simulink library "IIT_Genoa_Intan_HDL_blocks"  (R2020a)
settings: Solver=VariableStepAuto  StartTime=0.0  StopTime=10.0  RelTol=1e-3
libraries: simulink x93, hdlsllib x68
(part 1 of 3)
settings Model: Creator=diflo  LastModifiedBy=diflo

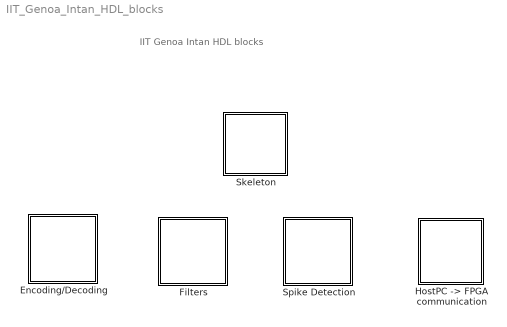
== system IIT_Genoa_Intan_HDL_blocks ==
  note: IIT Genoa Intan HDL blocks
  Encoding/Decoding : Subsystem
  Filters : Subsystem
  "HostPC -> FPGA communication" : Subsystem
  Skeleton : Subsystem
  Spike Detection : Subsystem

== system IIT_Genoa_Intan_HDL_blocks/Encoding//Decoding ==
  input_interpret_store_retrieve : Subsystem
      mask DialogControl DescGroupVar Prompt: Decoding subsystem
      mask DialogControl DescTextVar Prompt: This subsystem interprets the retrieved data from the Finite State Machine of the Intan RHS by assigning a specific value according to the data type.
      mask Display:
      | color('white'); port_label('input',1,'FIFO_data_in')
      | color('white'); port_label('input',2,'FIFO_write_to')
      | color('white'); port_label('input',3,'read_output_data_input_interpret_store_retrieve')
      | color('white'); port_label('input',4,'data_stream_enable')
      | color('white'); port_label('output',1,'InputState')
      | color('white'); port_label('output',2,'output_data_input_interpret_store_retrieve')
      | color('white'); port_label('output',3,'output_data_to_process')
      | color('white'); port_label('output',4,'address_output_data_to_process')
  output_interpret_collect_output : Subsystem
      mask DialogControl DescGroupVar Prompt: Encoding subsystem
      mask DialogControl DescTextVar Prompt: This subsystem reconstructs the logic of the dataflow in order to send the data to the Host PC.
      mask Display:
      | color('white'); port_label('input',1,'FIFO_data_in')
      | color('white'); port_label('input',2,'FIFO_write_to')
      | color('white'); port_label('input',3,'InputState')
      | color('white'); port_label('input',4,'data_stream_enable')
      | color('white'); port_label('input',5,'output_data_input_interpret_store_retrieve')
      | color('white'); port_label('input',6,'filter_output_or_spike')
      | color('white'); port_label('output',1,'comp_data_out_valid')
      | color('white'); port_label('output',2,'comp_data_out')
      | color('white'); port_label('output',3,'read_filter_output_or_spike')
      | color('white'); port_label('output',4,'OutputState')
      | color('white'); port_label('output',5,'read_output_data_input_interpret_store_retrieve')

== system IIT_Genoa_Intan_HDL_blocks/Filters ==
  Butter_1st_HP : Subsystem  mask{s1=0.969531252908746199, a21=-0.939062505817492399}
      mask DialogControl DescGroupVar Prompt: Direct Form II - Butterworth 1st Order HP filter
      mask DialogControl DescTextVar Prompt: Butterworth 1st order highpass filtering logic. The filter is fully serial implemented with a custom architecture according to the logic of the input dataflow from the Finite State Machine of the Intan RHS.
      mask DialogControl Container3 Prompt: Filter coefficients
      mask Display:
      | color('white'); port_label('input',1,'output_data_to_process')
      | color('white'); port_label('input',2,'InputState')
      | color('white'); port_label('input',3,'address_output_data_to_process')
      | color('white'); port_label('input',4,'read_filter_output_or_spike')
      | color('white'); port_label('output',1,'filter_output')
      | color('white'); port_label('output',2,'filter_writing_address')
      | color('white'); port_label('output',3,'filter_writing_enable')
      | color('white'); port_label('output',4,'filter_output_or_spike')
  Butter_2nd_HP : Subsystem  mask{s1=0.956543225556876764, a21=-1.9111970674260732, a31=0.914975834801433852, b21=-2}
      mask DialogControl DescGroupVar Prompt: Direct Form II - Butterworth 2nd Order HP filter
      mask DialogControl DescTextVar Prompt: Butterworth 2nd order highpass filtering logic. The filter is fully serial implemented with a custom architecture according to the logic of the input dataflow from the Finite State Machine of the Intan RHS.
      mask DialogControl ParameterGroupVar Prompt: Filter coefficients
      mask Display:
      | color('white'); port_label('input',1,'output_data_to_process')
      | color('white'); port_label('input',2,'InputState')
      | color('white'); port_label('input',3,'address_output_data_to_process')
      | color('white'); port_label('input',4,'read_filter_output_or_spike')
      | color('white'); port_label('output',1,'filter_output')
      | color('white'); port_label('output',2,'filter_writing_address')
      | color('white'); port_label('output',3,'filter_writing_enable')
      | color('white'); port_label('output',4,'filter_output_or_spike')

== system IIT_Genoa_Intan_HDL_blocks/HostPC -> FPGA communication ==
  interpret_pipe_in : Subsystem  TreatAsAtomicUnit=on
      mask DialogControl DescGroupVar Prompt: Pipe in interpret
      mask DialogControl DescTextVar Prompt: This subsystem interprets the configuration file loaded by the GUI running in the Host PC. It is possible to communicate a single value of threshold and refractory period for all the channels.
      mask Display:
      | color('white'); port_label('input',1,'pipe_in_data')
      | color('white'); port_label('output',1,'pipe_in_threshold')
      | color('white'); port_label('output',2,'pipe_in_refractory')

== system IIT_Genoa_Intan_HDL_blocks/Skeleton ==
  cust_architecture : Subsystem
      mask DialogControl DescGroupVar Prompt: Custom Architecture Skeleton
      mask DialogControl DescTextVar Prompt: High level skeleton of the custom architecture. The entire algorithm must be developed inside this subsystem.
      mask Display:
      | color('white'); port_label('input',1,'FIFO_data_in')
      | color('white'); port_label('input',2,'FIFO_write_to')
      | color('white'); port_label('input',3,'data_stream_enable')
      | color('white'); port_label('input',4,'pipe_in_data')
      | color('white'); port_label('input',5,'pipe_in_en')
      | color('white'); port_label('input',6,'pipe_out_read')
      | color('white'); port_label('input',7,'cfg')
      | color('white'); port_label('output',1,'comp_data_out')
      | color('white'); port_label('output',2,'comp_data_out_valid')
      | color('white'); port_label('output',3,'trig_stim')
      | color('white'); port_label('output',4,'computing')
      | color('white'); port_label('output',5,'pipe_out_data')
      | color('white'); port_label('output',6,'status')

== system IIT_Genoa_Intan_HDL_blocks/Spike Detection ==
  General : Subsystem
  Sample Thresholding : Subsystem
  Sample Trhesholding pipe in : Subsystem

== system IIT_Genoa_Intan_HDL_blocks/Encoding//Decoding/input_interpret_store_retrieve ==
  note: data sent to Output
  note: data sent for processing
  note: address sent for processing
  note: reading address
      | from output
  FIFO_data_in : Inport
  FIFO_write_to : Inport  Port=2
  read_output_data_input_interpret_store_retrieve : Inport  Port=3
  data_stream_enable : Inport  Port=4
  InputStateMachine : Stateflow chart  TreatAsAtomicUnit=on
  Interpret_to_RAM_input : Subsystem
  store_and_retrieve_input : Subsystem
  InputState : Outport
  output_data_input_interpret_store_retrieve : Outport  Port=2
  output_data_to_process : Outport  Port=3
  address_output_data_to_process : Outport  Port=4
  wires:
  Interpret_to_RAM_input/4(write address) -> store_and_retrieve_input/3(wr_address)
  Interpret_to_RAM_input/5(wr_en) -> store_and_retrieve_input/4(wr_en)
  InputStateMachine/1(InputState) -> store_and_retrieve_input/5(InputState), InputState/1, Interpret_to_RAM_input/3(InputState)  "InputState"
  store_and_retrieve_input/1(read_from_storage_value) -> output_data_input_interpret_store_retrieve/1
  Interpret_to_RAM_input/2(inc_source_device) -> InputStateMachine/4(inc_source_device_MSB)
  Interpret_to_RAM_input/1(device_output) -> InputStateMachine/3(channel_0_19)
  Interpret_to_RAM_input/3(wr_din) -> store_and_retrieve_input/2(wr_din)
  FIFO_data_in/1 -> InputStateMachine/1(FIFO_data_in), Interpret_to_RAM_input/1(FIFO_data_in)
  FIFO_write_to/1 -> Interpret_to_RAM_input/2(FIFO_write_to), InputStateMachine/2(FIFO_write_to)
  read_output_data_input_interpret_store_retrieve/1 -> store_and_retrieve_input/1(read address)
  data_stream_enable/1 -> Interpret_to_RAM_input/4(data_stream_enable)
  store_and_retrieve_input/3(read_from_porcessing_addr) -> address_output_data_to_process/1
  store_and_retrieve_input/2(current_value) -> output_data_to_process/1

== system IIT_Genoa_Intan_HDL_blocks/Encoding//Decoding/output_interpret_collect_output ==
  FIFO_data_in : Inport
  FIFO_write_to : Inport  Port=2
  InputState : Inport  Port=3
  data_stream_enable : Inport  Port=4
  output_data_input_interpret_store_retrieve : Inport  Port=5
  filter_output_or_spike : Inport  Port=6
  collect_output : Subsystem
  output_interpret : Subsystem
  comp_data_out_valid : Outport
  comp_data_out : Outport  Port=2
  read_filter_output_or_spike : Outport  Port=3
  OutputState : Outport  Port=4
  read_output_data_input_interpret_store_retrieve : Outport  Port=5
  wires:
  FIFO_data_in/1 -> collect_output/1(FIFO_data_in)
  output_interpret/1(OutputState) -> OutputState/1, collect_output/4(OutputState)
  FIFO_write_to/1 -> collect_output/2(FIFO_write_to)
  collect_output/2(comp_data_out) -> comp_data_out/1
  output_interpret/2(rd_enable) -> collect_output/5(rd_enable)
  output_interpret/3(read_output_data_input_interpret_store_retrieve) -> read_output_data_input_interpret_store_retrieve/1, collect_output/6(rd_address)
  collect_output/1(comp_data_out_valid) -> comp_data_out_valid/1
  output_data_input_interpret_store_retrieve/1 -> collect_output/7(read_from_storage_value)
  collect_output/3(rd_address_bit_set_AC_during_DC) -> read_filter_output_or_spike/1
  filter_output_or_spike/1 -> collect_output/8(rd_dout)
  data_stream_enable/1 -> output_interpret/1(data_stream_enable)
  InputState/1 -> output_interpret/2(InputState), collect_output/3(InputState)

== system IIT_Genoa_Intan_HDL_blocks/Filters/Butter_1st_HP ==
  output_data_to_process : Inport
  InputState : Inport  Port=2
  address_output_data_to_process : Inport  Port=3
  read_filter_output_or_spike : Inport  Port=4
  ProcessedData_storage : hdlsllib/HDL RAMs/Dual Port RAM  ram_size=9
      settings: SourceProductBaseCode=SL
  Subsystem : Subsystem
  Terminator1 : Terminator
  filter_output : Outport
  filter_writing_address : Outport  Port=2
  filter_writing_enable : Outport  Port=3
  filter_output_or_spike : Outport  Port=4
  wires:
  ProcessedData_storage/1 -> Terminator1/1
  ProcessedData_storage/2 -> filter_output_or_spike/1  "filtered_sample"
  read_filter_output_or_spike/1 -> ProcessedData_storage/4
  Subsystem/1(filter_output) -> filter_output/1, ProcessedData_storage/1
  Subsystem/2(filter_writing_address) -> filter_writing_address/1, ProcessedData_storage/2
  output_data_to_process/1 -> Subsystem/1(output_data_to_process)
  InputState/1 -> Subsystem/2(InputState)
  address_output_data_to_process/1 -> Subsystem/3(address_output_data_to_process)
  Subsystem/3(filter_writing_enable) -> filter_writing_enable/1, ProcessedData_storage/3

== system IIT_Genoa_Intan_HDL_blocks/Filters/Butter_2nd_HP ==
  output_data_to_process : Inport
  InputState : Inport  Port=2
  address_output_data_to_process : Inport  Port=3
  read_filter_output_or_spike : Inport  Port=4
  ProcessedData_storage : hdlsllib/HDL RAMs/Dual Port RAM  ram_size=9
      settings: SourceProductBaseCode=SL
  Terminator7 : Terminator
  filtering : Subsystem
  filter_output : Outport
  filter_writing_address : Outport  Port=2
  filter_writing_enable : Outport  Port=3
  filter_output_or_spike : Outport  Port=4
  wires:
  filtering/2(filter_writing_address) -> filter_writing_address/1, ProcessedData_storage/2
  filtering/3(filter_writing_enable) -> filter_writing_enable/1, ProcessedData_storage/3
  InputState/1 -> filtering/2(InputState)
  ProcessedData_storage/1 -> Terminator7/1
  read_filter_output_or_spike/1 -> ProcessedData_storage/4
  filtering/1(filter_output) -> filter_output/1, ProcessedData_storage/1
  output_data_to_process/1 -> filtering/1(output_data_to_process)
  ProcessedData_storage/2 -> filter_output_or_spike/1
  address_output_data_to_process/1 -> filtering/3(address_output_data_to_process)

== system IIT_Genoa_Intan_HDL_blocks/HostPC -> FPGA communication/interpret_pipe_in ==
  pipe_in_data : Inport
  pipe_in_refractory : Subsystem
  pipe_in_th : Subsystem
  threshold : Outport
  refractory : Outport  Port=2
  wires:
  pipe_in_data/1 -> pipe_in_th/1(value_from_pipe_in), pipe_in_refractory/1(value_from_pipe_in)
  pipe_in_refractory/1(refractory) -> refractory/1
  pipe_in_th/1(th) -> threshold/1

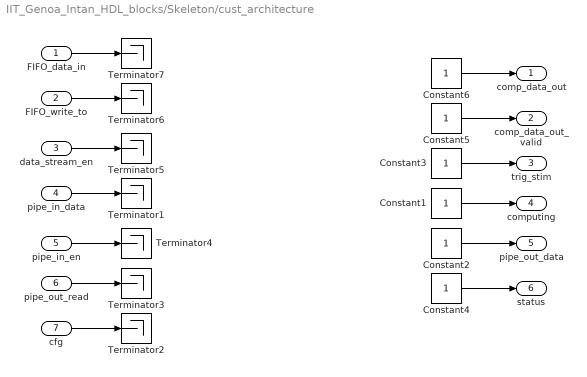
== system IIT_Genoa_Intan_HDL_blocks/Skeleton/cust_architecture ==
  FIFO_data_in : Inport
  FIFO_write_to : Inport  Port=2
  data_stream_en : Inport  Port=3
  pipe_in_data : Inport  Port=4
  pipe_in_en : Inport  Port=5
  pipe_out_read : Inport  Port=6
  cfg : Inport  Port=7
  Constant{1..6} (6 alike) : Constant  OutDataTypeStr=uint16  SampleTime=-1
  Terminator{1..7} (7 alike) : Terminator
  comp_data_out : Outport  VectorParamsAs1DForOutWhenUnconnected=off
  comp_data_out_valid : Outport  Port=2  OutDataTypeStr=boolean  VectorParamsAs1DForOutWhenUnconnected=off
  trig_stim : Outport  Port=3  VectorParamsAs1DForOutWhenUnconnected=off
  computing : Outport  Port=4  VectorParamsAs1DForOutWhenUnconnected=off
  pipe_out_data : Outport  Port=5  VectorParamsAs1DForOutWhenUnconnected=off
  status : Outport  Port=6  VectorParamsAs1DForOutWhenUnconnected=off
  wires:
  Constant3/1 -> trig_stim/1
  Constant1/1 -> computing/1
  Constant2/1 -> pipe_out_data/1
  Constant4/1 -> status/1
  cfg/1 -> Terminator2/1
  pipe_out_read/1 -> Terminator3/1
  pipe_in_en/1 -> Terminator4/1
  data_stream_en/1 -> Terminator5/1
  FIFO_write_to/1 -> Terminator6/1
  pipe_in_data/1 -> Terminator1/1
  FIFO_data_in/1 -> Terminator7/1
  Constant5/1 -> comp_data_out_valid/1
  Constant6/1 -> comp_data_out/1

== system IIT_Genoa_Intan_HDL_blocks/Spike Detection/General ==
  processing_output_logic : Subsystem
      mask DialogControl DescGroupVar Prompt: Output logic Filter/Spike Detection
      mask DialogControl DescTextVar Prompt: This subsystem is needed in order to send to the Host PC at the right time the filter outputs and the detected spikes
      mask Display:
      | color('white'); port_label('input',1,'OutputState')
      | color('white'); port_label('input',2,'filter_output')
      | color('white'); port_label('input',3,'spike')
      | color('white'); port_label('output',1,'to_output_interpret_collect_output')
  refractory_period : Subsystem  mask{refractory=0}
      mask prompts: refractory "Refractory period (samples)"
      mask DialogControl DescGroupVar Prompt: Refractory period
      mask DialogControl DescTextVar Prompt: Subsystem to compute the refractory period.
      mask Display:
      | color('white'); port_label('input',1,'filter_writing_enable')
      | color('white'); port_label('input',2,'spike_check')
      | color('white'); port_label('input',3,'filter_writing_address')
      | color('white'); port_label('input',4,'read_filter_output_or_spike')
      | color('white'); port_label('output',1,'refractory_check')
      | color('white'); port_label('output',2,'spike')
  refractory_period_pipe_in : Subsystem  AncestorBlock=IIT_Genoa_Intan_HDL_blocks/refractory_period
      mask DialogControl DescGroupVar Prompt: Refractory period (pipe in)
      mask DialogControl DescTextVar Prompt: Subsystem to compute the refractory period. The refractory period can be selected loading a configuration file from the GUI running in the Host PC in order to change in real time the value. This subsystem allows to set a single refractory period for all the channels.
      mask Display:
      | color('white'); port_label('input',1,'filter_writing_enable')
      | color('white'); port_label('input',2,'spike_check')
      | color('white'); port_label('input',3,'filter_writing_address')
      | color('white'); port_label('input',4,'read_filter_output_or_spike')
      | color('white'); port_label('input',5,'pipe_in_refractory')
      | color('white'); port_label('output',1,'refractory_check')
      | color('white'); port_label('output',2,'spike')
  spike_check : Subsystem
      mask DialogControl DescGroupVar Prompt: Spike check
      mask DialogControl DescTextVar Prompt: The ouput of this subsystem is 1 if both the refractory period condition and the amplitude check are TRUE, thus, a spike is detected and its timestamp stored.
      mask Display:
      | color('white'); port_label('input',1,'detection_check')
      | color('white'); port_label('input',2,'refractory_check')
      | color('white'); port_label('output',1,'spike_check')

== system IIT_Genoa_Intan_HDL_blocks/Spike Detection/Sample Thresholding ==
  HardThreshold : Subsystem  mask{th=0}
      mask prompts: th "Threshold (µV)"
      mask DialogControl DescGroupVar Prompt: Hard Threshold
      mask DialogControl DescTextVar Prompt: This subsystem computes a spike detection based on the identification of a sample in the signal below a set threshold. It detects as a potential each sample below threshold
      mask DialogControl ParameterGroupVar Prompt: Spike Detection Parametes
      mask Display:
      | color('white'); port_label('input',1,'filter_output')
      | color('white'); port_label('output',1,'detection_check')
  LocalMaxima : Subsystem  mask{th=0}
      mask prompts: th "Threshold (µV)"
      mask DialogControl DescGroupVar Prompt: Hard Threshold Local Maxima
      mask DialogControl DescTextVar Prompt: This subsystem computes a spike detection based on the identification of a peak in the signal below a set threshold. It takes into account the samples at time t, t-1 and t-2 to detect a potential negative peak below threshold.
      mask DialogControl Container Prompt: Spike detection parameters
      mask Display:
      | color('white'); port_label('input',1,'filter_output')
      | color('white'); port_label('input',2,'filter_writing_enable')
      | color('white'); port_label('input',3,'filter_writing_address')
      | color('white'); port_label('output',1,'detection_check')

== system IIT_Genoa_Intan_HDL_blocks/Spike Detection/Sample Trhesholding pipe in ==
  HardThreshold_pipein : Subsystem  AncestorBlock=IIT_Genoa_Intan_HDL_blocks/HardThreshold
      mask DialogControl DescGroupVar Prompt: Hard Threshold
      mask DialogControl DescTextVar Prompt: This subsystem computes a spike detection based on the identification of a sample in the signal below a set threshold. It detects as a potential each sample below threshold. The threshold can be selected loading a configuration file from the GUI running in the Host PC in order to change in real time the value. This subsystem allows to set a single threshold for all the channels.
      mask Display:
      | color('white'); port_label('input',1,'filter_output')
      | color('white'); port_label('input',2,'pipe_in_threshold')
      | color('white'); port_label('output',1,'detection_check')
  LocalMaxima_pipein : Subsystem  AncestorBlock=IIT_Genoa_Intan_HDL_blocks/LocalMaxima
      mask DialogControl DescGroupVar Prompt: Hard Threshold Local Maxima (pipe in)
      mask DialogControl DescTextVar Prompt: This subsystem computes a spike detection based on the identification of a peak in the signal below a set threshold. It takes into account the samples at time t, t-1 and t-2 to detect a potential negative peak below threshold. The threshold can be selected loading a configuration file from the GUI running in the Host PC in order to change in real time the value. This subsystem allows to set a single threshold for all the channels.
      mask Display:
      | color('white'); port_label('input',1,'filter_output')
      | color('white'); port_label('input',2,'filter_writing_enable')
      | color('white'); port_label('input',3,'filter_writing_address')
      | color('white'); port_label('input',4,'pipe_in_threshold')
      | color('white'); port_label('output',1,'detection_check')

== system IIT_Genoa_Intan_HDL_blocks/Encoding//Decoding/input_interpret_store_retrieve/Interpret_to_RAM_input ==
  note: These subsystems identify the sources of the incoming data (amplifier --> source_device and channel number) and
      | determine the address to be associated to the current data for the RAM storage. This statement is valid for all the kind of
      | data except for the magic number and the timestamp that are directly sent to a different RAM in the Output section
  FIFO_data_in : Inport
  FIFO_write_to : Inport  Port=2
  InputState : Inport  Port=3
  data_stream_enable : Inport  Port=4
  RAM address definition : Subsystem
  interpret incoming data : Subsystem
  device_output : Outport
  inc_source_device : Outport  Port=2
  wr_din : Outport  Port=3
  write address : Outport  Port=4
  wr_en : Outport  Port=5
  wires:
  interpret incoming data/4(source_channel_0_159) -> RAM address definition/3(source_channel_0_159)
  interpret incoming data/2(inc_source_device) -> inc_source_device/1
  interpret incoming data/1(source_device) -> RAM address definition/4(source_device)
  data_stream_enable/1 -> interpret incoming data/3(data_stream_enable)
  RAM address definition/3(write_enable_6to15) -> wr_en/1  "wr_en"
  interpret incoming data/3(device_output) -> device_output/1
  InputState/1 -> RAM address definition/2(InputState), interpret incoming data/2(InputState)
  interpret incoming data/5(converter_cnt) -> RAM address definition/5(converter_cnt)
  FIFO_write_to/1 -> RAM address definition/6(write_to), interpret incoming data/1(FIFO_write_to)
  FIFO_data_in/1 -> RAM address definition/1(DataIn)
  RAM address definition/2(wr_addr) -> write address/1  "write address"
  RAM address definition/1(wr_din) -> wr_din/1  "wr_din"

== system IIT_Genoa_Intan_HDL_blocks/Encoding//Decoding/input_interpret_store_retrieve/store_and_retrieve_input ==
  note: Two dual-port RAM for storage and processing
  note: current data
  note: data sent to Output
  note: data sent for processing
  note: this memory is for synchronizing the current value and
      | the read_from_porcessing_addr since to ouput a value
      | the dual port RAM needs a single clock
  note: current data
  note: reading address
      | from output
  note: address sent for processing
  note: writing address
  read address : Inport
  wr_din : Inport  Port=2
  wr_address : Inport  Port=3
  wr_en : Inport  Port=4
  InputState : Inport  Port=5
  Compare To Constant : simulink/Logic and Bit Operations/Compare To Constant  relop===  const=7  OutDataTypeStr=boolean
  Delay1 : Delay  DelayLength=1  InitialCondition=0
  Terminator : Terminator
  Terminator6 : Terminator
  input_storage : hdlsllib/HDL RAMs/Dual Port RAM  ram_size=9
      settings: SourceProductBaseCode=SL
  input_storage_for_processing : hdlsllib/HDL RAMs/Dual Port RAM  ram_size=9
      settings: SourceProductBaseCode=SL
  read_from_storage_value : Outport
  current_value : Outport  Port=2
  read_from_porcessing_addr : Outport  Port=3
  wires:
  wr_en/1 -> input_storage/3
  InputState/1 -> Compare To Constant/1
  Compare To Constant/1 -> input_storage_for_processing/3
  input_storage_for_processing/2 -> current_value/1  "current value"
  Delay1/1 -> read_from_porcessing_addr/1, input_storage_for_processing/4  "read from porcessing addr"
  input_storage/1 -> Terminator/1
  wr_address/1 -> Delay1/1, input_storage_for_processing/2, input_storage/2
  wr_din/1 -> input_storage_for_processing/1, input_storage/1
  input_storage/2 -> read_from_storage_value/1  "read_from_storage"
  input_storage_for_processing/1 -> Terminator6/1
  read address/1 -> input_storage/4

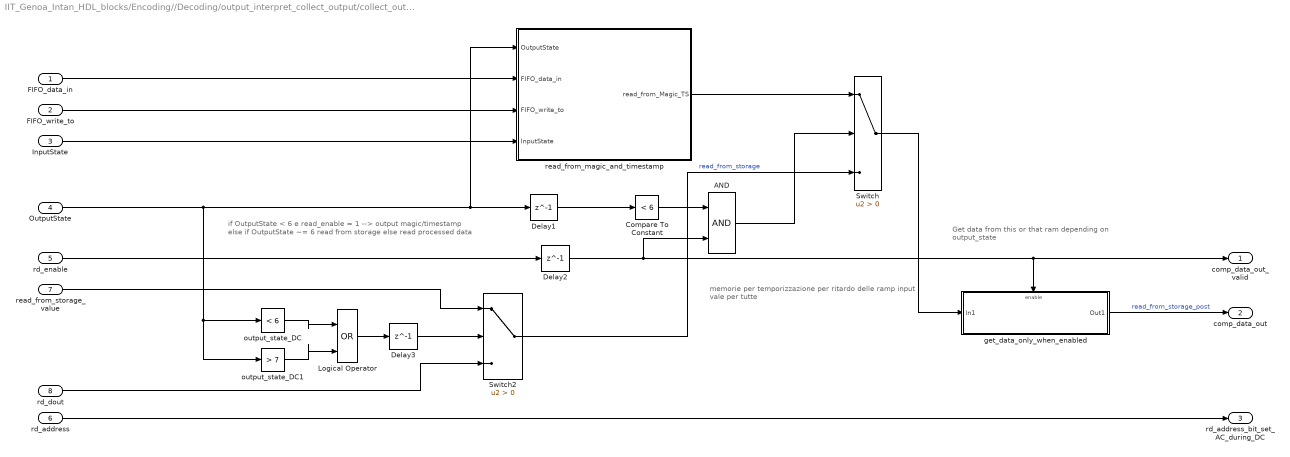
== system IIT_Genoa_Intan_HDL_blocks/Encoding//Decoding/output_interpret_collect_output/collect_output ==
  note: if OutputState < 6 e read_enable = 1 --> output magic/timestamp
      | else if OutputState ~= 6 read from storage
      | else read processed data
  note: memorie per temporizzazione per ritardo delle ramp input
      | vale per tutte
  note: Get data from this or that ram depending on output_state
  FIFO_data_in : Inport
  FIFO_write_to : Inport  Port=2
  InputState : Inport  Port=3
  OutputState : Inport  Port=4
  rd_enable : Inport  Port=5
  rd_address : Inport  Port=6
  read_from_storage_value : Inport  Port=7
  rd_dout : Inport  Port=8
  AND : Logic  IconShape=distinctive  AllPortsSameDT=off  OutDataTypeStr=boolean
  Compare To Constant : simulink/Logic and Bit Operations/Compare To Constant  relop=<  const=6  OutDataTypeStr=boolean
  Delay1 : Delay  DelayLength=1  InitialCondition=0
  Delay2 : Delay  DelayLength=1  InitialCondition=0
  Delay3 : Delay  DelayLength=1  InitialCondition=0
  Logical Operator : Logic  Operator=OR  IconShape=distinctive  AllPortsSameDT=off  OutDataTypeStr=boolean
  Switch : Switch  Criteria=u2 > Threshold
  Switch2 : Switch  Criteria=u2 > Threshold
  get_data_only_when_enabled : Subsystem  TreatAsAtomicUnit=on
  output_state_DC : simulink/Logic and Bit Operations/Compare To Constant  relop=<  const=6  OutDataTypeStr=boolean
  output_state_DC1 : simulink/Logic and Bit Operations/Compare To Constant  relop=>  const=7  OutDataTypeStr=boolean
  read_from_magic_and_timestamp : Subsystem
  comp_data_out_valid : Outport
  comp_data_out : Outport  Port=2
  rd_address_bit_set_AC_during_DC : Outport  Port=3
  wires:
  get_data_only_when_enabled/1(Out1) -> comp_data_out/1  "read_from_storage_post"
  FIFO_data_in/1 -> read_from_magic_and_timestamp/2(FIFO_data_in)
  read_from_storage_value/1 -> Switch2/1
  Delay1/1 -> Compare To Constant/1
  Delay2/1 -> AND/2, comp_data_out_valid/1, get_data_only_when_enabled/Enable
  Switch/1 -> get_data_only_when_enabled/1(In1)
  AND/1 -> Switch/2
  Switch2/1 -> Switch/3  "read_from_storage"
  Compare To Constant/1 -> AND/1
  read_from_magic_and_timestamp/1(read_from_Magic_TS) -> Switch/1
  rd_address/1 -> rd_address_bit_set_AC_during_DC/1
  rd_dout/1 -> Switch2/3
  rd_enable/1 -> Delay2/1
  FIFO_write_to/1 -> read_from_magic_and_timestamp/3(FIFO_write_to)
  InputState/1 -> read_from_magic_and_timestamp/4(InputState)
  OutputState/1 -> output_state_DC1/1, output_state_DC/1, Delay1/1, read_from_magic_and_timestamp/1(OutputState)
  output_state_DC1/1 -> Logical Operator/2
  output_state_DC/1 -> Logical Operator/1
  Logical Operator/1 -> Delay3/1
  Delay3/1 -> Switch2/2

== system IIT_Genoa_Intan_HDL_blocks/Encoding//Decoding/output_interpret_collect_output/output_interpret ==
  note: if InputState == 8 I have processed all the 20 channels (16ch + 4aux)
      | and I start with the output encoding
  data_stream_enable : Inport
  InputState : Inport  Port=2
  Interpret_to_RAM_output : Subsystem
  OutputStateMachine : Stateflow chart  TreatAsAtomicUnit=on
  OutputState : Outport
  rd_enable : Outport  Port=2
  read_output_data_input_interpret_store_retrieve : Outport  Port=3
  wires:
  OutputStateMachine/1(OutputState) -> OutputState/1, Interpret_to_RAM_output/1(OutputState)  "OutputState"
  Interpret_to_RAM_output/1(rd_enable) -> rd_enable/1
  data_stream_enable/1 -> Interpret_to_RAM_output/2(data_stream_en)
  InputState/1 -> OutputStateMachine/1(input_state)
  Interpret_to_RAM_output/2(read address) -> read_output_data_input_interpret_store_retrieve/1

== system IIT_Genoa_Intan_HDL_blocks/Filters/Butter_1st_HP/Subsystem ==
  output_data_to_process : Inport
  InputState : Inport  Port=2
  address_output_data_to_process : Inport  Port=3
  Memory2 : Memory  InheritSampleTime=on
  Memory3 : Memory  InheritSampleTime=on
  Memory5 : Memory  InheritSampleTime=on
  PreviousData_storage : hdlsllib/HDL RAMs/Dual Port RAM  ram_size=9
      settings: SourceProductBaseCode=SL
  Terminator8 : Terminator
  input_state_AC : simulink/Logic and Bit Operations/Compare To Constant  relop===  const=7  OutDataTypeStr=boolean
  one_pole_IIR : Subsystem
  filter_output : Outport
  filter_writing_address : Outport  Port=2
  filter_writing_enable : Outport  Port=3
  wires:
  Memory5/1 -> filter_writing_address/1, PreviousData_storage/2  "write porcessing addr = read from storage addr +1"
  address_output_data_to_process/1 -> PreviousData_storage/4, Memory5/1
  input_state_AC/1 -> Memory2/1  "read from porcessing"
  Memory3/1 -> input_state_AC/1
  one_pole_IIR/2(new_previous_sample) -> PreviousData_storage/1  "new_previous_sample"
  PreviousData_storage/1 -> Terminator8/1
  Memory2/1 -> filter_writing_enable/1, PreviousData_storage/3  "write en"
  PreviousData_storage/2 -> one_pole_IIR/2(previous_sample)  "previous_sample"
  one_pole_IIR/1(filter_output) -> filter_output/1  "filter_output"
  InputState/1 -> Memory3/1
  output_data_to_process/1 -> one_pole_IIR/1(output_data_to_process)

== system IIT_Genoa_Intan_HDL_blocks/Filters/Butter_2nd_HP/filtering ==
  note: this memory is to guarantee that the input is already stored
  note: Note: If a read operation occurs simultaneously at the same address
      | as a write operation, old data appears at the read output port (rd_dout).
  output_data_to_process : Inport
  InputState : Inport  Port=2
  address_output_data_to_process : Inport  Port=3
  Delay : Delay  DelayLength=1  InitialCondition=0
  Delay1 : Delay  DelayLength=1  InitialCondition=0
  Delay2 : Delay  DelayLength=1  InitialCondition=0
  Delay3 : Delay  DelayLength=3  InitialCondition=0
  Delay4 : Delay  DelayLength=3  InitialCondition=0
  Delay5 : Delay  InitialCondition=0
  Delay6 : Delay  InitialCondition=0
  Mux : Mux  Inputs=2
  PreviousData1_storage : hdlsllib/HDL RAMs/Dual Port RAM  ram_size=9
      settings: SourceProductBaseCode=SL
  PreviousData2_storage : hdlsllib/HDL RAMs/Dual Port RAM  ram_size=9
      settings: SourceProductBaseCode=SL
  Terminator2 : Terminator
  Terminator8 : Terminator
  input_state_AC : simulink/Logic and Bit Operations/Compare To Constant  relop===  const=7  OutDataTypeStr=boolean
  two_pole_IIR : Subsystem
  filter_output : Outport
  filter_writing_address : Outport  Port=2
  filter_writing_enable : Outport  Port=3
  wires:
  address_output_data_to_process/1 -> Delay2/1, PreviousData2_storage/4, PreviousData1_storage/4
  PreviousData1_storage/2 -> PreviousData2_storage/1, Mux/1  "previous_sample"
  Delay2/1 -> PreviousData2_storage/2, Delay5/1  "new_previous_sample"
  output_data_to_process/1 -> two_pole_IIR/1(output_data_to_process)
  Delay5/1 -> Delay3/1, PreviousData1_storage/2
  two_pole_IIR/2(new_previous_sample) -> PreviousData1_storage/1  "new_previous_sample"
  Delay1/1 -> Delay6/1, PreviousData2_storage/3  "write en"
  PreviousData1_storage/1 -> Terminator8/1
  Delay6/1 -> Delay4/1, PreviousData1_storage/3
  InputState/1 -> Delay/1
  PreviousData2_storage/1 -> Terminator2/1
  Delay/1 -> input_state_AC/1
  PreviousData2_storage/2 -> Mux/2  "previous_sample"
  input_state_AC/1 -> Delay1/1  "read from porcessing"
  Mux/1 -> two_pole_IIR/2(previous_sample)
  two_pole_IIR/1(filter_output) -> filter_output/1  "filter_output"
  Delay4/1 -> filter_writing_enable/1
  Delay3/1 -> filter_writing_address/1

== system IIT_Genoa_Intan_HDL_blocks/HostPC -> FPGA communication/interpret_pipe_in/pipe_in_refractory ==
  value_from_pipe_in : Inport
  Bit Slice : hdlsllib/Logic and Bit Operations/Bit Slice  lidx=1  ridx=0
      settings: SourceProductBaseCode=SL
  Compare To Constant : simulink/Logic and Bit Operations/Compare To Constant  relop===  const=1  OutDataTypeStr=boolean
  Constant : Constant  Value=0  OutDataTypeStr=uint16  SampleTime=-1
  Delay1 : Delay  DelayLength=1  InitialCondition=0
  Detect Change1 : simulink/Logic and Bit Operations/Detect Change  vinit=0  OutDataTypeStr=boolean
  Logical Operator1 : Logic  IconShape=distinctive  AllPortsSameDT=off  OutDataTypeStr=boolean
  Terminator : Terminator
  refractory_RAM : hdlsllib/HDL RAMs/Dual Port RAM  ram_size=2
      settings: SourceProductBaseCode=SL
  refractory : Outport
  wires:
  refractory_RAM/1 -> Terminator/1
  refractory_RAM/2 -> refractory/1
  Constant/1 -> Bit Slice/1
  Bit Slice/1 -> refractory_RAM/4, refractory_RAM/2
  Logical Operator1/1 -> refractory_RAM/3
  Delay1/1 -> Compare To Constant/1
  Detect Change1/1 -> Logical Operator1/1
  Compare To Constant/1 -> Logical Operator1/2
  value_from_pipe_in/1 -> Delay1/1, refractory_RAM/1, Detect Change1/1

== system IIT_Genoa_Intan_HDL_blocks/HostPC -> FPGA communication/interpret_pipe_in/pipe_in_th ==
  value_from_pipe_in : Inport
  Bit Slice : hdlsllib/Logic and Bit Operations/Bit Slice  lidx=1  ridx=0
      settings: SourceProductBaseCode=SL
  Compare To Constant : simulink/Logic and Bit Operations/Compare To Constant  relop===  const=0  OutDataTypeStr=boolean
  Constant : Constant  OutDataTypeStr=uint16  SampleTime=-1
  Delay1 : Delay  DelayLength=1  InitialCondition=0
  Detect Change1 : simulink/Logic and Bit Operations/Detect Change  vinit=0  OutDataTypeStr=boolean
  Logical Operator1 : Logic  IconShape=distinctive  AllPortsSameDT=off  OutDataTypeStr=boolean
  Terminator : Terminator
  refractory_RAM : hdlsllib/HDL RAMs/Dual Port RAM  ram_size=2
      settings: SourceProductBaseCode=SL
  th : Outport
  wires:
  refractory_RAM/1 -> Terminator/1
  refractory_RAM/2 -> th/1
  Constant/1 -> Bit Slice/1
  Bit Slice/1 -> refractory_RAM/4, refractory_RAM/2
  Logical Operator1/1 -> refractory_RAM/3
  Delay1/1 -> Compare To Constant/1
  Detect Change1/1 -> Logical Operator1/1
  Compare To Constant/1 -> Logical Operator1/2
  value_from_pipe_in/1 -> Delay1/1, refractory_RAM/1, Detect Change1/1

== system IIT_Genoa_Intan_HDL_blocks/Spike Detection/General/processing_output_logic ==
  OutputState : Inport
  filter_output : Inport  Port=2
  spike : Inport  Port=3
  Delay : Delay  DelayLength=1  InitialCondition=0
  Switch : Switch  Criteria=u2 > Threshold  Threshold=6
  to_output_interpret_collect_output : Outport
  wires:
  Switch/1 -> to_output_interpret_collect_output/1
  filter_output/1 -> Switch/1
  OutputState/1 -> Delay/1
  Delay/1 -> Switch/2
  spike/1 -> Switch/3

== system IIT_Genoa_Intan_HDL_blocks/Spike Detection/General/refractory_period ==
  filter_writing_enable : Inport
  spike_check : Inport  Port=2
  filter_writing_address : Inport  Port=3
  read_filter_output_or_spike : Inport  Port=4
  Constant : Constant  OutDataTypeStr=uint16  SampleTime=-1
  Constant1 : Constant  Value=0  OutDataTypeStr=uint16  SampleTime=-1
  Delay : Delay  DelayLength=1  InitialCondition=0
  HDL Counter : hdlsllib/Sources/HDL Counter  CountType=Free running  CountInit=0  CountStep=1  CountMax=2^32  CountFromType=Initial value  CountFrom=0  CountResetPort=off  CountLoadPort=off  CountEnbPort=on  CountDirPort=off  CountDataType=Unsigned  CountWordLen=32  CountFracLen=0  CountSampTime=1
  Logical Operator : Logic  IconShape=distinctive  AllPortsSameDT=off  OutDataTypeStr=boolean
  Sum : Sum  Inputs=+-
  Switch : Switch  Criteria=u2 > Threshold
  Terminator2 : Terminator
  Terminator3 : Terminator
  rd_addr_check : simulink/Logic and Bit Operations/Compare To Constant  relop===  const=1  OutDataTypeStr=boolean
  refractory_period : simulink/Logic and Bit Operations/Compare To Constant  relop=>=  const=refractory  OutDataTypeStr=boolean
  spikes : hdlsllib/HDL RAMs/Dual Port RAM  ram_size=9
      settings: SourceProductBaseCode=SL
  timestamp_before : hdlsllib/HDL RAMs/Dual Port RAM  ram_size=9
      settings: SourceProductBaseCode=SL
  refractory_check : Outport
  spike : Outport  Port=2
  wires:
  timestamp_before/1 -> Terminator2/1
  Delay/1 -> spikes/2, timestamp_before/2
  spikes/2 -> spike/1
  filter_writing_address/1 -> Delay/1, timestamp_before/4
  spike_check/1 -> Switch/2, timestamp_before/3
  timestamp_before/2 -> Sum/2
  read_filter_output_or_spike/1 -> rd_addr_check/1, spikes/4
  spikes/1 -> Terminator3/1
  Sum/1 -> refractory_period/1
  filter_writing_enable/1 -> spikes/3, Logical Operator/2  "read from porcessing"
  refractory_period/1 -> Logical Operator/1
  Logical Operator/1 -> refractory_check/1
  rd_addr_check/1 -> HDL Counter/1  "read from porcessing"
  HDL Counter/1 -> timestamp_before/1, Sum/1
  Constant/1 -> Switch/1
  Switch/1 -> spikes/1
  Constant1/1 -> Switch/3

== system IIT_Genoa_Intan_HDL_blocks/Spike Detection/General/refractory_period_pipe_in ==
  filter_writing_enable : Inport
  spike_check : Inport  Port=2
  filter_writing_address : Inport  Port=3
  read_filter_output_or_spike : Inport  Port=4
  pipe_in_refractory : Inport  Port=5
  Constant : Constant  OutDataTypeStr=uint16  SampleTime=-1
  Constant1 : Constant  Value=0  OutDataTypeStr=uint16  SampleTime=-1
  Delay : Delay  DelayLength=1  InitialCondition=0
  HDL Counter : hdlsllib/Sources/HDL Counter  CountType=Free running  CountInit=0  CountStep=1  CountMax=2^32  CountFromType=Initial value  CountFrom=0  CountResetPort=off  CountLoadPort=off  CountEnbPort=on  CountDirPort=off  CountDataType=Unsigned  CountWordLen=32  CountFracLen=0  CountSampTime=1
  Logical Operator : Logic  IconShape=distinctive  AllPortsSameDT=off  OutDataTypeStr=boolean
  Relational Operator : RelationalOperator  Operator=<  OutDataTypeStr=boolean  RndMeth=Simplest
  Sum : Sum  Inputs=+-
  Switch : Switch  Criteria=u2 > Threshold
  Terminator2 : Terminator
  Terminator3 : Terminator
  rd_addr_check : simulink/Logic and Bit Operations/Compare To Constant  relop===  const=1  OutDataTypeStr=boolean
  spikes : hdlsllib/HDL RAMs/Dual Port RAM  ram_size=9
      settings: SourceProductBaseCode=SL
  timestamp_before : hdlsllib/HDL RAMs/Dual Port RAM  ram_size=9
      settings: SourceProductBaseCode=SL
  refractory_check : Outport
  spike : Outport  Port=2
  wires:
  timestamp_before/1 -> Terminator2/1
  Delay/1 -> spikes/2, timestamp_before/2
  spikes/2 -> spike/1
  filter_writing_address/1 -> Delay/1, timestamp_before/4
  spike_check/1 -> Switch/2, timestamp_before/3
  timestamp_before/2 -> Sum/2
  read_filter_output_or_spike/1 -> rd_addr_check/1, spikes/4
  spikes/1 -> Terminator3/1
  Sum/1 -> Relational Operator/1
  filter_writing_enable/1 -> spikes/3, Logical Operator/2  "read from porcessing"
  Relational Operator/1 -> Logical Operator/1
  Logical Operator/1 -> refractory_check/1
  rd_addr_check/1 -> HDL Counter/1  "read from porcessing"
  HDL Counter/1 -> timestamp_before/1, Sum/1
  Constant/1 -> Switch/1
  Switch/1 -> spikes/1
  Constant1/1 -> Switch/3
  pipe_in_refractory/1 -> Relational Operator/2

== system IIT_Genoa_Intan_HDL_blocks/Spike Detection/General/spike_check ==
  detection_check : Inport
  refractory_check : Inport  Port=2
  Logical Operator : Logic  IconShape=distinctive  AllPortsSameDT=off  OutDataTypeStr=boolean
  spike_check : Outport
  wires:
  refractory_check/1 -> Logical Operator/2
  detection_check/1 -> Logical Operator/1
  Logical Operator/1 -> spike_check/1

== system IIT_Genoa_Intan_HDL_blocks/Spike Detection/Sample Thresholding/HardThreshold ==
  filter_output : Inport
  threshold : simulink/Logic and Bit Operations/Compare To Constant  relop=<  const=(th/(0.195))+32768  OutDataTypeStr=boolean
  detection_check : Outport
  wires:
  filter_output/1 -> threshold/1
  threshold/1 -> detection_check/1  "read from porcessing"

== system IIT_Genoa_Intan_HDL_blocks/Spike Detection/Sample Thresholding/LocalMaxima ==
  filter_output : Inport
  filter_writing_enable : Inport  Port=2
  filter_writing_address : Inport  Port=3
  Delay1 : Delay  DelayLength=1  InitialCondition=0
  Delay2 : Delay  DelayLength=1  InitialCondition=0
  Logical Operator1 : Logic  Inputs=3  IconShape=distinctive  AllPortsSameDT=off  OutDataTypeStr=boolean
  Terminator1 : Terminator
  Terminator2 : Terminator
  check_t-1 : RelationalOperator  Operator=<  OutDataTypeStr=boolean  RndMeth=Simplest
  check_t-2 : RelationalOperator  Operator=<  OutDataTypeStr=boolean  RndMeth=Simplest
  sample_t-1 : hdlsllib/HDL RAMs/Dual Port RAM  ram_size=9
      settings: SourceProductBaseCode=SL
  sample_t-2 : hdlsllib/HDL RAMs/Dual Port RAM  ram_size=9
      settings: SourceProductBaseCode=SL
  threshold : simulink/Logic and Bit Operations/Compare To Constant  relop=<  const=(th/(0.195))+32768  OutDataTypeStr=boolean
  detection_check : Outport
  wires:
  threshold/1 -> Logical Operator1/1
  sample_t-1/2 -> sample_t-2/1, check_t-2/1, check_t-1/1, threshold/1
  filter_output/1 -> sample_t-1/1, check_t-2/2
  check_t-2/1 -> Logical Operator1/3
  check_t-1/1 -> Logical Operator1/2
  sample_t-2/1 -> Terminator1/1
  sample_t-2/2 -> check_t-1/2
  sample_t-1/1 -> Terminator2/1
  Logical Operator1/1 -> detection_check/1
  filter_writing_enable/1 -> sample_t-2/3, sample_t-1/3
  filter_writing_address/1 -> sample_t-2/4, Delay2/1, Delay1/1, sample_t-1/4
  Delay2/1 -> sample_t-2/2
  Delay1/1 -> sample_t-1/2

== system IIT_Genoa_Intan_HDL_blocks/Spike Detection/Sample Trhesholding pipe in/HardThreshold_pipein ==
  filter_output : Inport
  pipe_in_threshold : Inport  Port=2
  Relational Operator : RelationalOperator  Operator=<  OutDataTypeStr=boolean  RndMeth=Simplest
  detection_check : Outport
  wires:
  filter_output/1 -> Relational Operator/1
  Relational Operator/1 -> detection_check/1  "read from porcessing"
  pipe_in_threshold/1 -> Relational Operator/2

== system IIT_Genoa_Intan_HDL_blocks/Spike Detection/Sample Trhesholding pipe in/LocalMaxima_pipein ==
  filter_output : Inport
  filter_writing_enable : Inport  Port=2
  filter_writing_address : Inport  Port=3
  pipe_in_data : Inport  Port=4
  Delay1 : Delay  DelayLength=1  InitialCondition=0
  Delay2 : Delay  DelayLength=1  InitialCondition=0
  Logical Operator1 : Logic  Inputs=3  IconShape=distinctive  AllPortsSameDT=off  OutDataTypeStr=boolean
  Relational Operator : RelationalOperator  Operator=<  OutDataTypeStr=boolean  RndMeth=Simplest
  Terminator1 : Terminator
  Terminator2 : Terminator
  check_t-1 : RelationalOperator  Operator=<  OutDataTypeStr=boolean  RndMeth=Simplest
  check_t-2 : RelationalOperator  Operator=<  OutDataTypeStr=boolean  RndMeth=Simplest
  sample_t-1 : hdlsllib/HDL RAMs/Dual Port RAM  ram_size=9
      settings: SourceProductBaseCode=SL
  sample_t-2 : hdlsllib/HDL RAMs/Dual Port RAM  ram_size=9
      settings: SourceProductBaseCode=SL
  detection_check : Outport
  wires:
  Relational Operator/1 -> Logical Operator1/1
  sample_t-1/2 -> sample_t-2/1, Relational Operator/1, check_t-2/1, check_t-1/1
  filter_output/1 -> sample_t-1/1, check_t-2/2
  check_t-2/1 -> Logical Operator1/3
  check_t-1/1 -> Logical Operator1/2
  sample_t-2/1 -> Terminator1/1
  sample_t-2/2 -> check_t-1/2
  sample_t-1/1 -> Terminator2/1
  Logical Operator1/1 -> detection_check/1
  filter_writing_enable/1 -> sample_t-2/3, sample_t-1/3
  filter_writing_address/1 -> sample_t-2/4, Delay2/1, Delay1/1, sample_t-1/4
  Delay2/1 -> sample_t-2/2
  Delay1/1 -> sample_t-1/2
  pipe_in_data/1 -> Relational Operator/2

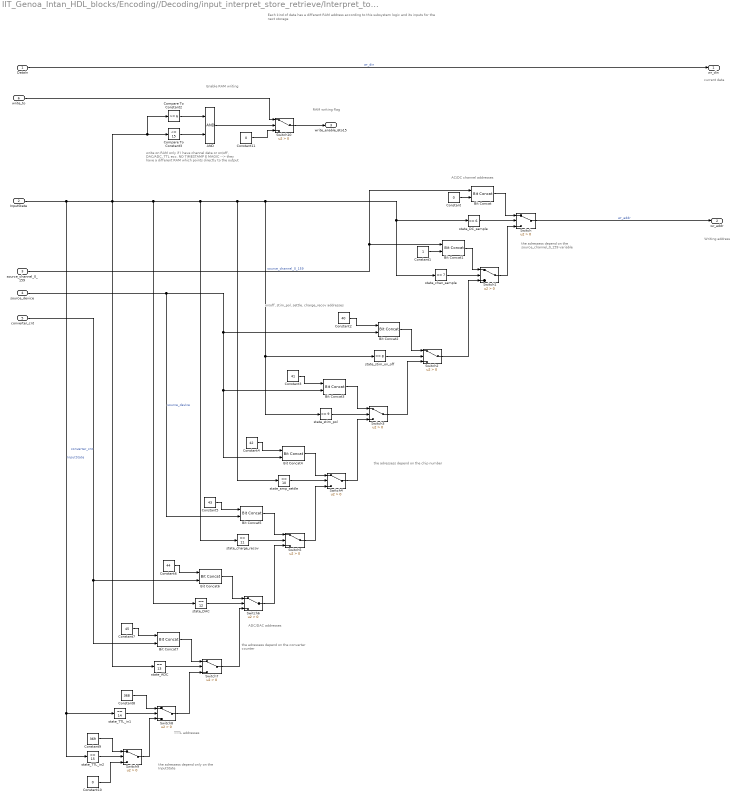
== system IIT_Genoa_Intan_HDL_blocks/Encoding//Decoding/input_interpret_store_retrieve/Interpret_to_RAM_input/RAM address definition ==
  note: the adressess depend on the chip number
  note: Each kind of data has a different RAM
      | address according to this subsystem logic
      | and its inputs for the next storage
  note: AC/DC channel addresses
  note: Writing address
  note: current data
  note: RAM writing flag
  note: write on RAM only if I have channel data or on/off,
      | DAC/ADC, TTL ecc.
      | NO TIMESTAMP E MAGIC --> they have a different
      | RAM which points directly to the output
  note: on/off, stim_pol, settle, charge_recov addresses
  note: ADC/DAC addresses
  note: TTTL addresses
  note: the adressess depend on the converter
      | counter
  note: the adressess depend only on the
      | InputState
  note: the adressess depend on the
      | source_channel_0_159 variable
  note: Enable RAM writing
  DataIn : Inport
  InputState : Inport  Port=2
  source_channel_0_159 : Inport  Port=3
  source_device : Inport  Port=4
  converter_cnt : Inport  Port=5
  write_to : Inport  Port=6  OutDataTypeStr=boolean
  AND : Logic  IconShape=distinctive  AllPortsSameDT=off  OutDataTypeStr=boolean
  Bit Concat{,1..7} (8 alike) : hdlsllib/Logic and Bit Operations/Bit Concat  numInputs=2
  Compare To Constant2 : simulink/Logic and Bit Operations/Compare To Constant  relop=>=  const=6  OutDataTypeStr=boolean
  Compare To Constant3 : simulink/Logic and Bit Operations/Compare To Constant  relop=<=  const=15  OutDataTypeStr=boolean
  Constant : Constant  Value=0  OutDataTypeStr=boolean  SampleTime=-1
  Constant1 : Constant  OutDataTypeStr=boolean  SampleTime=-1
  Constant10 : Constant  Value=0  OutDataTypeStr=fixdt(0,9)  SampleTime=-1
  Constant11 : Constant  Value=0  OutDataTypeStr=boolean  SampleTime=-1
  Constant2 : Constant  Value=40  OutDataTypeStr=fixdt(0,6)  SampleTime=-1
  Constant3 : Constant  Value=41  OutDataTypeStr=fixdt(0,6)  SampleTime=-1
  Constant4 : Constant  Value=42  OutDataTypeStr=fixdt(0,6)  SampleTime=-1
  Constant5 : Constant  Value=43  OutDataTypeStr=fixdt(0,6)  SampleTime=-1
  Constant6 : Constant  Value=44  OutDataTypeStr=fixdt(0,6)  SampleTime=-1
  Constant7 : Constant  Value=45  OutDataTypeStr=fixdt(0,6)  SampleTime=-1
  Constant8 : Constant  Value=368  OutDataTypeStr=fixdt(0,9)  SampleTime=-1
  Constant9 : Constant  Value=369  OutDataTypeStr=fixdt(0,9)  SampleTime=-1
  Switch{,1..10} (11 alike) : Switch  Criteria=u2 > Threshold
  state_ADC : simulink/Logic and Bit Operations/Compare To Constant  relop===  const=13  OutDataTypeStr=boolean
  state_DAC : simulink/Logic and Bit Operations/Compare To Constant  relop===  const=12  OutDataTypeStr=boolean
  state_DC_sample : simulink/Logic and Bit Operations/Compare To Constant  relop===  const=6  OutDataTypeStr=boolean
  state_TTL_in1 : simulink/Logic and Bit Operations/Compare To Constant  relop===  const=14  OutDataTypeStr=boolean
  state_TTL_in2 : simulink/Logic and Bit Operations/Compare To Constant  relop===  const=15  OutDataTypeStr=boolean
  state_amp_settle : simulink/Logic and Bit Operations/Compare To Constant  relop===  const=10  OutDataTypeStr=boolean
  state_chan_sample : simulink/Logic and Bit Operations/Compare To Constant  relop===  const=7  OutDataTypeStr=boolean
  state_charge_recov : simulink/Logic and Bit Operations/Compare To Constant  relop===  const=11  OutDataTypeStr=boolean
  state_stim_on_off : simulink/Logic and Bit Operations/Compare To Constant  relop===  const=8  OutDataTypeStr=boolean
  state_stim_pol : simulink/Logic and Bit Operations/Compare To Constant  relop===  const=9  OutDataTypeStr=boolean
  wr_din : Outport  VectorParamsAs1DForOutWhenUnconnected=off
  wr_addr : Outport  Port=2  OutDataTypeStr=fixdt(0,9,0)  VectorParamsAs1DForOutWhenUnconnected=off
  write_enable_6to15 : Outport  Port=3  OutDataTypeStr=boolean  VectorParamsAs1DForOutWhenUnconnected=off
  wires:
  state_DC_sample/1 -> Switch/2
  source_channel_0_159/1 -> Bit Concat1/1, Bit Concat/1  "source_channel_0_159"
  Constant/1 -> Bit Concat/2
  Bit Concat/1 -> Switch/1
  state_chan_sample/1 -> Switch1/2
  Constant1/1 -> Bit Concat1/2
  Bit Concat1/1 -> Switch1/1
  Switch1/1 -> Switch/3
  Switch/1 -> wr_addr/1  "wr_addr"
  Constant2/1 -> Bit Concat2/1
  Bit Concat2/1 -> Switch2/1
  state_stim_on_off/1 -> Switch2/2
  Switch2/1 -> Switch1/3
  Constant3/1 -> Bit Concat3/1
  state_stim_pol/1 -> Switch3/2
  Bit Concat3/1 -> Switch3/1
  Switch3/1 -> Switch2/3
  Constant4/1 -> Bit Concat4/1
  state_amp_settle/1 -> Switch4/2
  Bit Concat4/1 -> Switch4/1
  Switch4/1 -> Switch3/3
  Bit Concat5/1 -> Switch5/1
  state_charge_recov/1 -> Switch5/2
  Constant5/1 -> Bit Concat5/1
  source_device/1 -> Bit Concat5/2, Bit Concat4/2, Bit Concat3/2, Bit Concat2/2  "source_device"
  Switch5/1 -> Switch4/3
  Bit Concat6/1 -> Switch6/1
  state_DAC/1 -> Switch6/2
  Constant6/1 -> Bit Concat6/1
  Switch6/1 -> Switch5/3
  converter_cnt/1 -> Bit Concat7/2, Bit Concat6/2  "converter_cnt"
  Bit Concat7/1 -> Switch7/1
  state_ADC/1 -> Switch7/2
  Constant7/1 -> Bit Concat7/1
  Switch7/1 -> Switch6/3
  state_TTL_in1/1 -> Switch8/2
  Constant8/1 -> Switch8/1
  Switch8/1 -> Switch7/3
  state_TTL_in2/1 -> Switch9/2
  Constant9/1 -> Switch9/1
  Switch9/1 -> Switch8/3
  Constant10/1 -> Switch9/3
  DataIn/1 -> wr_din/1  "wr_din"
  Compare To Constant3/1 -> AND/2
  InputState/1 -> state_TTL_in1/1, state_TTL_in2/1, state_ADC/1, state_DAC/1, state_charge_recov/1, state_amp_settle/1, state_stim_pol/1, state_stim_on_off/1, state_chan_sample/1, state_DC_sample/1, Compare To Constant2/1, Compare To Constant3/1  "InputState"
  AND/1 -> Switch10/2
  Switch10/1 -> write_enable_6to15/1
  write_to/1 -> Switch10/1
  Compare To Constant2/1 -> AND/1
  Constant11/1 -> Switch10/3
